simulink model "AM"  (R2017a)
settings: Solver=ode4  StartTime=0.0  StopTime=2  FixedStep=0.001  RelTol=1e-3
libraries: simulink_extras x6, dsparch4 x2
settings Model: Creator=carma  LastModifiedBy=carma

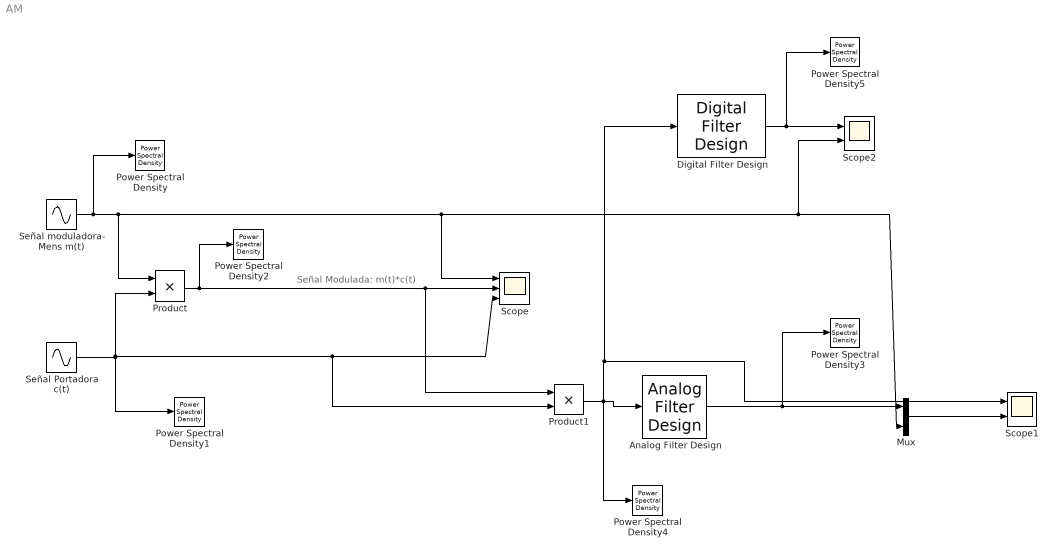
== system AM ==
  note: Señal Modulada: m(t)*c(t)
  Analog Filter Design : dsparch4/Analog Filter Design  method=Butterworth  filttype=Lowpass  N=8  Wlo=50  Whi=80  Rp=2  Rs=40
  Digital Filter Design : dsparch4/Digital Filter Design  mwdsp_browser_bugfix_var=off
  Mux : Mux  Inputs=2
  Power Spectral Density{,1..5} (6 alike) : simulink_extras/Additional Sinks/Power Spectral Density  npts=512  fftpts=1024  HowOften=64  sampleT=0.001
      settings: SourceProductName=Simulink  SourceProductBaseCode=SL
  Product : Product
  Product1 : Product
  Scope : Scope  NumInputPorts=3
  Scope1 : Scope  NumInputPorts=2
  Scope2 : Scope  NumInputPorts=2
  Señal Portadora c(t) : Sin  Amplitude=2  Frequency=500  SampleTime=0
  Señal moduladora- Mens m(t) : Sin  Amplitude=0.5  Frequency=50  SampleTime=0
  wires:
  Señal Portadora c(t)/1 -> Product1/2, Scope/3, Product/2, Power Spectral Density1/1
  Product/1 -> Power Spectral Density2/1, Product1/1, Scope/2
  Product1/1 -> Power Spectral Density4/1, Digital Filter Design/1, Scope1/1, Analog Filter Design/1
  Analog Filter Design/1 -> Mux/1, Power Spectral Density3/1
  Mux/1 -> Scope1/2
  Digital Filter Design/1 -> Power Spectral Density5/1, Scope2/1
  Señal moduladora- Mens m(t)/1 -> Power Spectral Density/1, Scope2/2, Mux/2, Scope/1, Product/1
